simulink model "morpho"  (R2016a)
settings: Solver=VariableStepAuto  StartTime=0.0  StopTime=1  RelTol=1e-3
undefined symbols (not defined in the file or in its folder): strel
libraries: visionsources x4, visionconversions x3, visionmorphops x2, visionutilities x1
settings Model: Creator=Shadhin  LastModifiedBy=Shadhin

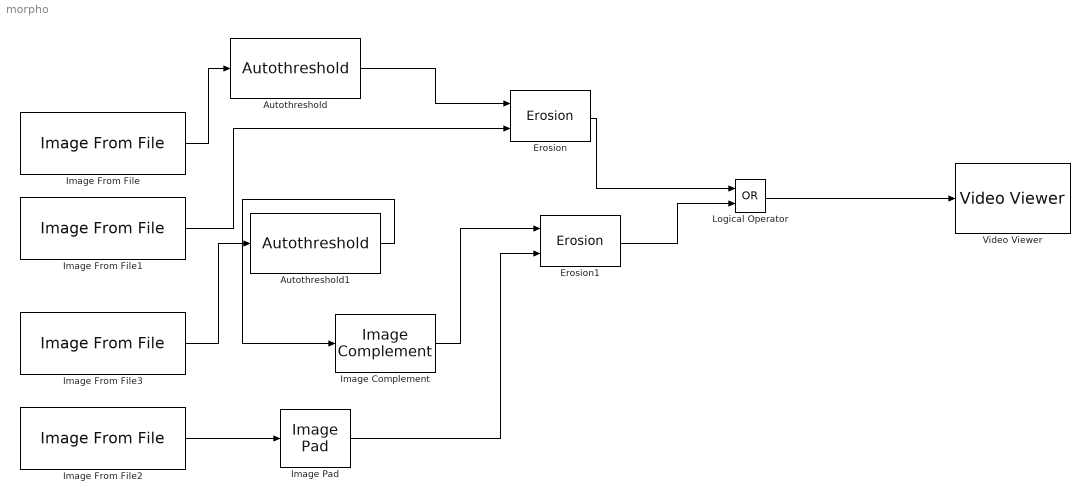
== system morpho ==
  Autothreshold : visionconversions/Autothreshold  operator=>  threshOut=off  effMetricOut=off  userDefinedRange=off  umin=0  umax=255  outOfRngOpt=Warn and saturate  scaleThreshold=on  scaleFactor=0.9  P1Mode=Specify word length  P1WordLength=32  P1FracLength=30  P2Mode=Specify word length  P2WordLength=32  P2FracLength=22  P3Mode=Specify word length  P3WordLength=32  P3FracLength=14  P4Mode=Binary point scaling  P4WordLength=32  P4FracLength=15  Q1Mode=Specify word length  Q1WordLength=32  Q1FracLength=16  EMMode=Specify word length  EMWordLength=16  EMFracLength=14  roundingMode=Floor  overflowMode=off
  Autothreshold1 : visionconversions/Autothreshold  operator=>  threshOut=off  effMetricOut=off  userDefinedRange=off  umin=0  umax=255  outOfRngOpt=Warn and saturate  scaleThreshold=on  scaleFactor=0.9  P1Mode=Specify word length  P1WordLength=32  P1FracLength=30  P2Mode=Specify word length  P2WordLength=32  P2FracLength=22  P3Mode=Specify word length  P3WordLength=32  P3FracLength=14  P4Mode=Binary point scaling  P4WordLength=32  P4FracLength=15  Q1Mode=Specify word length  Q1WordLength=32  Q1FracLength=16  EMMode=Specify word length  EMWordLength=16  EMFracLength=14  roundingMode=Floor  overflowMode=off
  Erosion : visionmorphops/Erosion  nhoodsrc=Input port  strel=strel('square',4)
  Erosion1 : visionmorphops/Erosion  nhoodsrc=Input port  strel=strel('square',4)
  Image Complement : visionconversions/Image Complement
  Image From File : visionsources/Image From File  Tag=vipblks_nd  FileName=E:\Education\4.2\Digital Image Processing\CharSet\N1.jpg  imagePorts=One multidimensional signal  Ts=1  ImageDataType=Inherit from input image  Signed=on  WordLength=16  sdImageDataType=uint(8)  FractionLengthMode=User-defined  FractionLength=15  OutPortLabels=R|G|B
  Image From File1 : visionsources/Image From File  Tag=vipblks_nd  FileName=C:\Users\Shadhin\Downloads\Number Plate Extraction using MATLAB\code\templates\6.bmp  imagePorts=One multidimensional signal  Ts=1  ImageDataType=boolean  Signed=on  WordLength=16  sdImageDataType=uint(8)  FractionLengthMode=User-defined  FractionLength=15  OutPortLabels=R|G|B
  Image From File2 : visionsources/Image From File  Tag=vipblks_nd  FileName=C:\Users\Shadhin\Downloads\Number Plate Extraction using MATLAB\code\templates\6.bmp  imagePorts=One multidimensional signal  Ts=1  ImageDataType=boolean  Signed=on  WordLength=16  sdImageDataType=uint(8)  FractionLengthMode=User-defined  FractionLength=15  OutPortLabels=R|G|B
  Image From File3 : visionsources/Image From File  Tag=vipblks_nd  FileName=E:\Education\4.2\Digital Image Processing\CharSet\N1.jpg  imagePorts=One multidimensional signal  Ts=1  ImageDataType=Inherit from input image  Signed=on  WordLength=16  sdImageDataType=uint(8)  FractionLengthMode=User-defined  FractionLength=15  OutPortLabels=R|G|B
  Image Pad : visionutilities/Image Pad  method=Constant  valSrc=Specify via dialog  value=0  spec=Pad size  rowDirection=Both left and right  outRowsMode=User-specified  rowSize=2  outColSize=10  colDirection=Both top and bottom  outColsMode=User-specified  colSize=[2 3]  outRowSize=12  trunc_flag=None
  Logical Operator : Logic  Operator=OR
  Video Viewer : VideoViewer  FigPos=[1 726 1366 627]
  wires:
  Image From File1/1 -> Erosion/2
  Erosion/1 -> Logical Operator/1
  Erosion1/1 -> Logical Operator/2
  Image Complement/1 -> Erosion1/1
  Logical Operator/1 -> Video Viewer/1
  Image From File2/1 -> Image Pad/1
  Image Pad/1 -> Erosion1/2
  Image From File/1 -> Autothreshold/1
  Autothreshold/1 -> Erosion/1
  Image From File3/1 -> Autothreshold1/1
  Autothreshold1/1 -> Image Complement/1
